simulink model "PV_MEV"  (R2025a)
settings: Solver=VariableStepAuto  StartTime=0.0  StopTime=10.0  RelTol=1e-3
InitFcn:
  | init_paras
values from neighbouring files (symbols this model uses):
  C_PFC = 2600e-6    (= 0.0026)    [init_paras.m]
  chg_ctrl_par = [Icc Vcv V_hys T_hys Kp_v_chg Ki_v_chg Kp_i_chg Ki_i_chg Ts_chg D_max_chg t_chg_on k_chg]    [init_paras.m]
  chg_ev = [0 Icc]    [init_paras.m]
  chg_par = [L_chg Voc Rint Ts_chg I_SIGN t_chg_on]    [init_paras.m]
  D = struct('X', {}, 'ti', {}, 'ia', {}, 'tc', {}, 'irms', {}, 'thd', {}, 'trip', {}, 'ttrip', {})    [make_waveform_figs.m]    (also in run_benchmark.m = get_sig('D'))
  det_ema_alpha = 0.1    [init_paras.m]
  det_force = 0    [init_paras.m]
  det_hyst = 0.6    [init_paras.m]
  det_persist = 2    [init_paras.m]
  det_src = 0    [init_paras.m]
  det_t_arm = 0.58    [init_paras.m]
  det_thr = [0.5 0.5 0.5 0.5 0.5]    [init_paras.m]
  det_variant_onehot = double(det_vlist == VARIANT_NAME)    [init_paras.m]
  ENABLE_HIL = 0    [init_paras.m]
  ENABLE_HIL_DET = 0    [init_paras.m]
  ENABLE_HIL_EST = 0    [init_paras.m]
  estimation_src = cfg_row.estimation_src    [init_paras.m]
  Fnom = 50    [init_paras.m]
  Fr_I = Fnom*2    (= 100)    [init_paras.m]
  grid_df = 0    [init_paras.m]
  grid_h5 = 0    [init_paras.m]
  grid_h7 = 0    [init_paras.m]
  grid_var_t0 = 0.7    [init_paras.m]
  hgq_fusion_alpha = [0.6704476522845647 0.7221651725151749 0.6446423751787858 0.41926421682656173]    [init_paras.m]
  hgq_min_ratio = single(0)    [init_paras.m]
  inj_channel = INJ.channel    [init_paras.m]
  inj_dwell = INJ.dwell    [init_paras.m]
  inj_shape = INJ.shape    [init_paras.m]
  inj_t_on = INJ.t_on    [init_paras.m]
  Ki_V = 80    [init_paras.m]
  Kp_I = 0.06    [init_paras.m]
  Kp_V = 0.25    [init_paras.m]
  Kr_I = 2.5    [init_paras.m]
  L_PFC = 600e-6    (= 0.0006)    [init_paras.m]
  Limit_V = 100    [init_paras.m]
  mit_t_ramp = 0.06    [init_paras.m]
  mitigation_mask = 0    [init_paras.m]
  mm_10cycle_points = mm_points_per_cycle * 10    (= 800)    [init_paras.m]
  mm_fund_freq = 50    [init_paras.m]
  mm_points_per_cycle = 80    [init_paras.m]
  R_bleed = 100e3    (= 100000)    [init_paras.m]
  R_pre = Ro*2    (= 44.44)    [init_paras.m]
  res_par = double(RES.par(:)'); end    [init_paras.m]
  RL_PFC = 20e-3    (= 0.02)    [init_paras.m]
  Ro = 22.22    [init_paras.m]
  t_pre_off = 0.30    (= 0.3)    [init_paras.m]
  Ts_chg = 10e-6    (= 1e-05)    [init_paras.m]
  Ts_Control = 1/Fc    [init_paras.m]
  Ts_Power = 50e-9    (= 5e-08)    [init_paras.m]    (also in run_benchmark.m = evalin('base','Ts_Power'))
  use_d_predict = cfg_row.use_d_predict    [init_paras.m]
  use_detector = 0    [init_paras.m]
  use_harmonic = cfg_row.use_harmonic    [init_paras.m]
  use_p_predict = cfg_row.use_p_predict    [init_paras.m]
  Vnom_ac = 240    [init_paras.m]
  vref_ev = [0 0]    [init_paras.m]
undefined symbols (not defined in the file or in its folder): D1, Delta, DiscIntNeverNeededParam
libraries: spsSeriesRLCBranchLib x17, spsMeanLib x16, MyLibrary x12, spsCurrentMeasurementLib x9, spsFourierLib x8, spsTHDLib x8, spsVoltageMeasurementLib x8, spsDiodeLib x7, simulink x7, pycoexlib x5, instrumentlib x4, spsPWMGeneratorDCDCLib x4
(part 5 of 7)

== system PV_MEV/PV System/DC DC Boost Converter ==
  note: 5 kHz - 500V
      | Boost Converter
  C1 : spsSeriesRLCBranchLib/Series RLC Branch  LConnTagsString=__new0  RConnTagsString=__new0  BranchType=C  Resistance=1.0  Inductance=1.0  SetiL0=off  InitialCurrent=0  Capacitance=12000e-06  Setx0=off  InitialVoltage=0  Measurements=None
  C2 : spsSeriesRLCBranchLib/Series RLC Branch  LConnTagsString=__new0  RConnTagsString=__new0  BranchType=C  Resistance=1.0  Inductance=1.0  SetiL0=off  InitialCurrent=0  Capacitance=12000e-06  Setx0=off  InitialVoltage=0  Measurements=None
  C3 : spsSeriesRLCBranchLib/Series RLC Branch  LConnTagsString=__new0  RConnTagsString=__new0  BranchType=C  Resistance=1.0  Inductance=1.0  SetiL0=off  InitialCurrent=0  Capacitance=100e-6  Setx0=off  InitialVoltage=0  Measurements=Branch voltage
  Deblock Converters : Step  Time=0.05  SampleTime=0
  Diode1 : spsDiodeLib/Diode  Ron=1e-4  Lon=0  Vf=0  IC=0  UseSnubber=off  Rs=inf  Cs=inf  Measurements=off
  Display : Display
  IGBT1 : spsIGBTLib/IGBT  Ron=0.001  Lon=0  Vf=0  Tf=0  Tt=0  IC=0  Rs=1e5  Cs=inf  Measurements=off
  L1 : spsSeriesRLCBranchLib/Series RLC Branch  LConnTagsString=__new0  RConnTagsString=__new0  BranchType=RL  Resistance=0.005  Inductance=5e-3  SetiL0=off  InitialCurrent=0  Capacitance=1e-6  Setx0=off  InitialVoltage=0  Measurements=None
  "MPPT Controller using  'Incremental Conductance + Integral Regulator'  technique " : Subsystem  mask(Boost Control - MPPT){fc=5000, T_MPPT=200e-6, Dinit=0.5}
      mask prompts: fc "PWM switching frequency (Hz)"; T_MPPT "Time window used by MPPT control (s)"; Dinit "Initial value of duty cycle"
  Product2 : Product  RndMeth=Zero
  "Vdc " : spsVoltageMeasurementLib/Voltage Measurement  Tag=PoWeRsYsTeMmEaSuReMeNt  PhasorSimulation=off  OutputType=Magnitude  PSBequivalent=0
  PV DC IN + : PMIOPort  Side=Left
  PV DC IN - : PMIOPort  Port=2  Side=Left
  BC DC OUT + : PMIOPort  Port=3  Side=Right
  BC DC MID : PMIOPort  Port=4  Side=Right
  BC DC OUT - : PMIOPort  Port=5  Side=Right
  tag scope: Vdc=global
  wires:
  Product2/1 -> IGBT1/1
  "Vdc "/1 -> Display/1, [Vdc]
  "MPPT Controller using  'Incremental Conductance + Integral Regulator'  technique "/1(Pulses) -> Product2/2
  Deblock Converters/1 -> Product2/1
  [V_PV] -> "MPPT Controller using  'Incremental Conductance + Integral Regulator'  technique "/1(V_PV)
  [I_PV] -> "MPPT Controller using  'Incremental Conductance + Integral Regulator'  technique "/2(I_PV)
  connections:
  Diode1/RConn1 -- "Vdc "/LConn1 -- C1/LConn1 -- BC DC OUT +/RConn1
  PV DC IN -/RConn1 -- C3/RConn1 -- IGBT1/RConn1 -- "Vdc "/LConn2 -- C2/RConn1 -- BC DC OUT -/RConn1
  L1/RConn1 -- Diode1/LConn1 -- IGBT1/LConn1
  C2/LConn1 -- C1/RConn1 -- BC DC MID/RConn1
  PV DC IN +/RConn1 -- C3/LConn1 -- L1/LConn1

== system PV_MEV/PV System/PV Enviroment ==
  Irradiance (W/m^2) : Display
  Irradiance Temp : SignalEditorBlockLib/Signal Editor  FileName=PVArrayGridData.mat  ActiveScenario=Ramp_up_down_Irradiance  ActiveSignal=Temp  IsBus=off  OutputBusObjectStr=Bus: BusObject  SampleTime=0  OutputAfterFinalValue=Extrapolation  Unit=inherit  PreserveSignalName=on  ApplySigPropsToAllScenarios=on  ApplySigPropsToAllSignals=off  SignalPropertySource=Dialog parameters
  Temperature (deg. C) : Display
  Ir : Outport
  Temp : Outport  Port=2
  wires:
  Irradiance Temp/1 -> Irradiance (W/m^2)/1, Ir/1
  ? -> Temperature (deg. C)/1, Temp/1

== system PV_MEV/PV System/PV Status ==
  m_PV : Inport
  Bus Selector : BusSelector  OutputSignals=V_PV,I_PV,I_diode,Irradiance (W/m2),Temperature (deg C)
  tag scope: I_PV=global, Idiode_PV=global, Ir=global, Temp=global, V_PV=global
  wires:
  Bus Selector/5 -> [Temp]  "<Temperature (deg C)>"
  Bus Selector/3 -> [Idiode_PV]  "<I_diode>"
  Bus Selector/2 -> [I_PV]  "<I_PV>"
  m_PV/1 -> Bus Selector/1
  Bus Selector/4 -> [Ir]  "<Irradiance (W/m2)>"
  Bus Selector/1 -> [V_PV]  "<V_PV>"

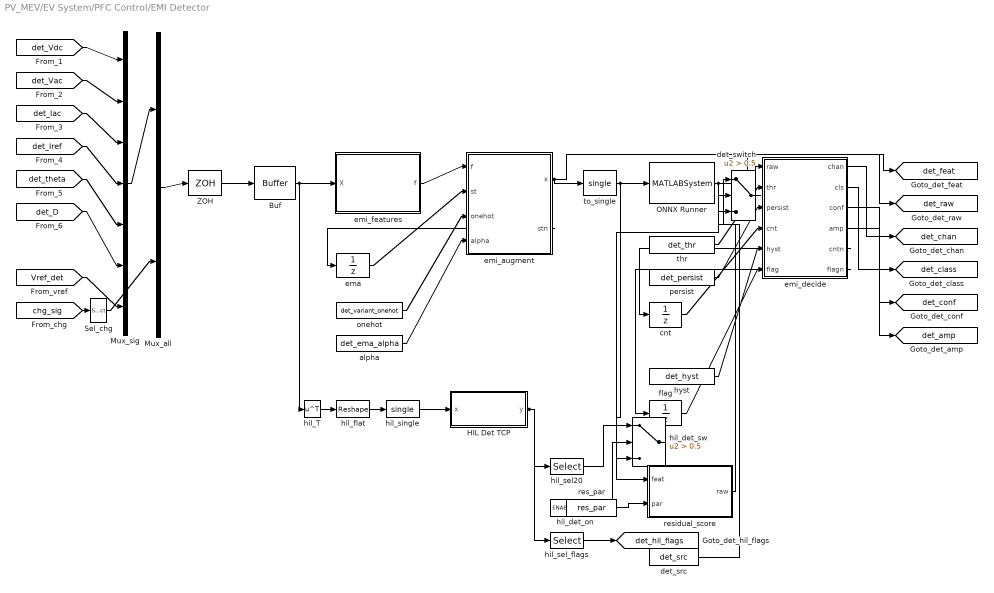
== system PV_MEV/EV System/PFC Control/EMI Detector ==
  Buf : Buffer  N=200
  HIL Det TCP : MATLAB Function  TreatAsAtomicUnit=on
  Mux_all : Mux  Inputs=2
  Mux_sig : Mux  Inputs=7
  ONNX Runner : MATLABSystem  System=OnnxRunner  ModelFile=/mnt/data6/playground/OLD_BRANCH/RL4EV/EMI_DET_FPGA/artifacts/detector.onnx  NumIn=48  NumOut=20  SampleTime=0.02
      mask Type: OnnxRunner
  Sel_chg : Selector  InputPortWidth=9  IndexOptions=Index vector (dialog)  Indices=[3 4 5 6 7]  OutputSizes=1
  ZOH : ZeroOrderHold  SampleTime=1e-4
  alpha : Constant  Value=det_ema_alpha
  cnt : UnitDelay  InitialCondition=zeros(1,5)  SampleTime=0.02  HasFrameUpgradeWarning=on
  det_src : Constant  Value=det_src
  det_switch : Switch  Criteria=u2 > Threshold  Threshold=0.5  SaturateOnIntegerOverflow=off  InputSameDT=off
  ema : UnitDelay  InitialCondition=zeros(1,49)  SampleTime=0.02  HasFrameUpgradeWarning=on
  emi_augment : MATLAB Function  TreatAsAtomicUnit=on
  emi_decide : MATLAB Function  TreatAsAtomicUnit=on
  emi_features : MATLAB Function  TreatAsAtomicUnit=on
  flag : UnitDelay  InitialCondition=zeros(1,5)  SampleTime=0.02  HasFrameUpgradeWarning=on
  hil_T : Math  Operator=transpose
  hil_det_on : Constant  Value=ENABLE_HIL_DET
  hil_det_sw : Switch  Criteria=u2 > Threshold  Threshold=0.5  SaturateOnIntegerOverflow=off  InputSameDT=off
  hil_flat : Reshape  OutputDimensionality=Row vector (2-D)
  hil_sel20 : Selector  InputPortWidth=21  IndexOptions=Index vector (dialog)  Indices=1:20  OutputSizes=1
  hil_sel_flags : Selector  InputPortWidth=21  IndexOptions=Index vector (dialog)  Indices=21  OutputSizes=1
  hil_single : DataTypeConversion  OutDataTypeStr=single  SaturateOnIntegerOverflow=off  RndMeth=Floor
  hyst : Constant  Value=det_hyst
  onehot : Constant  Value=det_variant_onehot
  persist : Constant  Value=det_persist
  res_par : Constant  Value=res_par
  residual_score : MATLAB Function  TreatAsAtomicUnit=on
  thr : Constant  Value=det_thr
  to_single : DataTypeConversion  OutDataTypeStr=single  SaturateOnIntegerOverflow=off  RndMeth=Floor
  tag scope: det_amp=global, det_chan=global, det_class=global, det_conf=global, det_feat=global, det_hil_flags=global, det_raw=global
  wires:
  [det_Vdc] -> Mux_sig/1
  [det_Vac] -> Mux_sig/2
  [det_Iac] -> Mux_sig/3
  [det_Iref] -> Mux_sig/4
  [det_theta] -> Mux_sig/5
  [det_D] -> Mux_sig/6
  [Vref_det] -> Mux_sig/7
  [chg_sig] -> Sel_chg/1
  Mux_sig/1 -> Mux_all/1
  Sel_chg/1 -> Mux_all/2
  Mux_all/1 -> ZOH/1
  ZOH/1 -> Buf/1
  Buf/1 -> emi_features/1(X), hil_T/1
  emi_features/1(f) -> emi_augment/1(f)
  ema/1 -> emi_augment/2(st)
  onehot/1 -> emi_augment/3(onehot)
  alpha/1 -> emi_augment/4(alpha)
  emi_augment/2(stn) -> ema/1
  emi_augment/1(x) -> to_single/1, [det_feat]
  to_single/1 -> ONNX Runner/1, residual_score/1(feat)
  ONNX Runner/1 -> [det_raw], hil_det_sw/3, det_switch/3
  thr/1 -> emi_decide/2(thr)
  persist/1 -> emi_decide/3(persist)
  cnt/1 -> emi_decide/4(cnt)
  hyst/1 -> emi_decide/5(hyst)
  flag/1 -> emi_decide/6(flag)
  emi_decide/5(cntn) -> cnt/1
  emi_decide/6(flagn) -> flag/1
  emi_decide/1(chan) -> [det_chan]
  emi_decide/2(cls) -> [det_class]
  emi_decide/3(conf) -> [det_conf]
  emi_decide/4(amp) -> [det_amp]
  hil_T/1 -> hil_flat/1
  hil_flat/1 -> hil_single/1
  hil_sel20/1 -> hil_det_sw/1
  hil_det_on/1 -> hil_det_sw/2
  hil_sel_flags/1 -> [det_hil_flags]
  hil_single/1 -> HIL Det TCP/1(x)
  HIL Det TCP/1(y) -> hil_sel20/1, hil_sel_flags/1
  res_par/1 -> residual_score/2(par)
  residual_score/1(raw) -> det_switch/1
  det_src/1 -> det_switch/2
  det_switch/1 -> emi_decide/1(raw)

== system PV_MEV/EV System/PFC Control/Enabled Subsystem ==
  Iac : Inport
  Data Type Conversion : DataTypeConversion  OutDataTypeStr=single  SaturateOnIntegerOverflow=off  RndMeth=Floor
  FFT Peak Hz : Display
  FFT Peak Receive : instrumentlib/TCP//IP Receive  Priority=20  Host=134.226.86.100  Port=5003  DataSize=[1, 1]  DataType=single  ASCIIFormatting=%f  Terminator=LF  CustomTerminator=10  ByteOrder=little-endian  EnableBlockingMode=on  Timeout=10  SampleTime=1/4000  SimulateUsing=Interpreted execution
  FFT TCP Send : instrumentlib/TCP//IP Send  Priority=-9  Host=134.226.86.100  Port=5002  ByteOrder=little-endian  EnableBlockingMode=on  Timeout=10  TransferDelay=off  SimulateUsing=Interpreted execution
  Scope1 : Scope  NumInputPorts=3
      settings: DataLoggingVariableName=ScopeData8  DataLoggingSaveFormat=Array
  TCP Sample Hold : ZeroOrderHold  SampleTime=1/4000
  TCP/IP Receive1 : instrumentlib/TCP//IP Receive  Priority=10  Host=134.226.86.100  Port=5001  DataSize=[1, 1]  DataType=single  ASCIIFormatting=%f  Terminator=LF  CustomTerminator=10  ByteOrder=little-endian  EnableBlockingMode=on  Timeout=10  SampleTime=1/4000  SimulateUsing=Interpreted execution
  TCP/IP Send1 : instrumentlib/TCP//IP Send  Priority=-10  Host=134.226.86.100  Port=5000  ByteOrder=little-endian  EnableBlockingMode=on  Timeout=10  TransferDelay=off  SimulateUsing=Interpreted execution
  wires:
  Data Type Conversion/1 -> Scope1/2, TCP/IP Send1/1, FFT TCP Send/1
  Iac/1 -> Scope1/1, TCP Sample Hold/1
  TCP Sample Hold/1 -> Data Type Conversion/1
  FFT Peak Receive/1 -> FFT Peak Hz/1
  TCP/IP Receive1/1 -> Scope1/3

== system PV_MEV/EV System/PFC Control/Half Cycle Model Prediction ==
  u : Inport
  Constant1 : Constant  Value=0.01
  Data Type Conversion : DataTypeConversion  SaturateOnIntegerOverflow=off  RndMeth=Floor
  Data Type Conversion1 : DataTypeConversion  SaturateOnIntegerOverflow=off  RndMeth=Floor
  Data Type Conversion2 : DataTypeConversion  SaturateOnIntegerOverflow=off  RndMeth=Floor
  Demux : Demux  Outputs=7
  MATLAB Function : MATLAB Function  TreatAsAtomicUnit=on
  MATLAB Function3 : MATLAB Function  TreatAsAtomicUnit=on
  Mux1 : Mux  Inputs=3
  Mux6 : Mux
  ONNX Model Predict : pycoexlib/ONNX Model Predict  ModelFile=/home/changhong/prj/finn_cli_fork/scripts/HIL/HarmonicAI_Simulation/Model_Training2/harmonic_brevitas_run_half_opt/brevitas_harmonic_mlp.onnx  ExecutionProviders=CPUExecutionProvider  InputTable={ 'input', 'float32', '', '2' }  OutputTable={ 'output', '', '' }  SampleTime=1/2000  InputDatatypes=float32  InputNumDims=2  InputPermutations=[]  OutputPermutations=[]  PythonCoexecutionBlockType=ONNXModelBlock  VariableOutputMaxSizes=[]
  Sampling1 : ZeroOrderHold  SampleTime=1/2000
  Transpose : Math  Operator=transpose
  u_buff : Buffer  N=40  V=39  OutputFrames=off
  amplitude : Outport
  phase : Outport  Port=2
  wires:
  Transpose/1 -> MATLAB Function/1(x)
  u_buff/1 -> Transpose/1
  u/1 -> Sampling1/1
  Mux1/1 -> phase/1
  Mux6/1 -> amplitude/1
  Data Type Conversion2/1 -> Demux/1
  MATLAB Function3/1(y_post) -> Data Type Conversion2/1
  Demux/1 -> Mux6/1
  Demux/2 -> Mux6/2
  Demux/3 -> Mux6/3
  Demux/4 -> Mux6/4
  Demux/5 -> Mux1/1
  Demux/6 -> Mux1/2
  Demux/7 -> Mux1/3
  MATLAB Function/2(A) -> MATLAB Function3/2(A_latest)
  Constant1/1 -> MATLAB Function3/3(alpha)
  Data Type Conversion1/1 -> MATLAB Function3/1(y_rel)
  ONNX Model Predict/1 -> Data Type Conversion1/1
  Data Type Conversion/1 -> ONNX Model Predict/1
  MATLAB Function/1(x_norm) -> Data Type Conversion/1
  Sampling1/1 -> u_buff/1

== system PV_MEV/EV System/PFC Control/One  Cycle Model Prediction ==
  u : Inport
  Constant1 : Constant
  Data Type Conversion : DataTypeConversion  SaturateOnIntegerOverflow=off  RndMeth=Floor
  Data Type Conversion1 : DataTypeConversion  SaturateOnIntegerOverflow=off  RndMeth=Floor
  Data Type Conversion2 : DataTypeConversion  SaturateOnIntegerOverflow=off  RndMeth=Floor
  Demux : Demux  Outputs=7
  HIL Est TCP : MATLAB Function  TreatAsAtomicUnit=on
  MATLAB Function : MATLAB Function  TreatAsAtomicUnit=on
  MATLAB Function3 : MATLAB Function  TreatAsAtomicUnit=on
  Mux1 : Mux  Inputs=3
  Mux6 : Mux
  ONNX Runner : MATLABSystem  System=OnnxRunner  ModelFile='D:/Prj/RL4EV/FFT_HGQ_BLS_FPGA/artifacts/harmonic_residual_bls_simulink.onnx'  NumIn=80  NumOut=8  SampleTime=1/(mm_fund_freq*mm_points_per_cycle)
      mask Type: OnnxRunner
  Sampling1 : ZeroOrderHold  SampleTime=1/(mm_fund_freq*mm_points_per_cycle)
  Transpose : Math  Operator=transpose
  hil_est_on : Constant  Value=ENABLE_HIL_EST
  hil_est_sw : Switch  Criteria=u2 > Threshold  Threshold=0.5  SaturateOnIntegerOverflow=off  InputSameDT=off
  hil_row : Reshape  OutputDimensionality=Row vector (2-D)
  hil_single : DataTypeConversion  OutDataTypeStr=single  SaturateOnIntegerOverflow=off  RndMeth=Floor
  u_buff : Buffer  N=mm_points_per_cycle  V=mm_sampling_overlap  OutputFrames=off
  amplitude : Outport
  phase : Outport  Port=2
  wires:
  Sampling1/1 -> u_buff/1
  MATLAB Function/1(x_norm) -> Data Type Conversion/1
  Data Type Conversion1/1 -> MATLAB Function3/1(y_encoded)
  Constant1/1 -> MATLAB Function3/3(ema_alpha)
  MATLAB Function/2(A) -> MATLAB Function3/2(window_peak)
  Demux/7 -> Mux1/3
  Demux/6 -> Mux1/2
  Demux/5 -> Mux1/1
  Demux/4 -> Mux6/4
  Demux/3 -> Mux6/3
  Demux/2 -> Mux6/2
  Demux/1 -> Mux6/1
  MATLAB Function3/1(y_post) -> Data Type Conversion2/1
  Data Type Conversion2/1 -> Demux/1
  Mux6/1 -> amplitude/1
  Mux1/1 -> phase/1
  u/1 -> Sampling1/1
  u_buff/1 -> Transpose/1
  Transpose/1 -> MATLAB Function/1(x), hil_single/1
  Data Type Conversion/1 -> ONNX Runner/1
  hil_single/1 -> hil_row/1
  hil_est_on/1 -> hil_est_sw/2
  ONNX Runner/1 -> hil_est_sw/3
  hil_est_sw/1 -> Data Type Conversion1/1
  hil_row/1 -> HIL Est TCP/1(x)
  HIL Est TCP/1(y) -> hil_est_sw/1

== system PV_MEV/EV System/PFC Control/PR2 ==
  Iref : Inport
  Iac : Inport  Port=2
  Gain : Gain  Gain=Kp
  Gain1 : Gain  Gain=Kr
  Second-Order Filter1 : spsSecondOrderFilterLib/Second-Order Filter  FilterType=Bandpass  Fo=Fr  Zeta=Zeta_I  Ts=Ts_Control  Initialize=off  Vac_Init="[0,  0,  60]"  Vdc_Init=0  PlotResponse=off  FreqRange=[0, 1000, 0.2]
  Sum1 : Sum  Inputs=|+-
  Sum2 : Sum  Inputs=|++
  D : Outport
  wires:
  Gain1/1 -> Second-Order Filter1/1
  Sum2/1 -> D/1
  Gain/1 -> Sum2/1
  Iac/1 -> Sum1/2
  Iref/1 -> Sum1/1
  Sum1/1 -> Gain1/1, Gain/1
  Second-Order Filter1/1 -> Sum2/2

== system PV_MEV/EV System/PFC Control/Speed Regulator2 ==
  note: Anti-windup mechanism: Method of conditionnal integration
      |
      | The integration is suspended if saturation occurs and the
      | control error is of the same sign as the control signal.
      |
      | [1] L.Rundqwist, "Anti-Reset Windup for PID Controllers," Ph.D. Thesis TRFT-1033,
      | Departement of Automatic Control, Lund Institute of Technology, Lund, Sweeden, 1991.
  Vref : Inport  PortDimensions=1
  Vmeas : Inport  Port=2  PortDimensions=1
  Ilim : Inport  Port=3
  Add : Sum  Inputs=+|-
  Compare To Zero : simulink/Logic and Bit Operations/Compare To Zero  relop=>  OutDataTypeStr=uint8  ZeroCross=off
  Compare To Zero1 : simulink/Logic and Bit Operations/Compare To Zero  relop=<  OutDataTypeStr=uint8  ZeroCross=off
  Constant : Constant  Value=0
  Discrete-Time Integrator : DiscreteIntegrator  IntegratorMethod=Integration: Trapezoidal  InitialCondition=Init  SampleTime=Ts  LimitOutput=on  UpperSaturationLimit=Limit_wreg  LowerSaturationLimit=-Limit_wreg  ShowStatePort=on  ICPrevOutput=DiscIntNeverNeededParam  ICPrevScaledInput=DiscIntNeverNeededParam
  Kp4 : Gain  Gain=Kp  SaturateOnIntegerOverflow=on  SampleTime=Ts  OutDataTypeStr=Inherit: Same as input  ParamDataTypeStr=Inherit: Same as input
  Kp5 : Gain  Gain=Ki  SaturateOnIntegerOverflow=on  SampleTime=Ts  OutDataTypeStr=Inherit: Same as input  ParamDataTypeStr=Inherit: Same as input
  Logical Operator : Logic  AllPortsSameDT=off  OutDataTypeStr=boolean
  Logical Operator1 : Logic  AllPortsSameDT=off  OutDataTypeStr=boolean
  Logical Operator2 : Logic  Operator=OR  AllPortsSameDT=off  OutDataTypeStr=boolean
  Relational Operator : RelationalOperator  OutDataTypeStr=boolean  InputSameDT=off
  Relational Operator1 : RelationalOperator  Operator=<=  OutDataTypeStr=boolean  InputSameDT=off
  SatDyn : simulink/Discontinuities/Saturation Dynamic  OutMin=[]  OutMax=[]  OutDataTypeStr=Inherit: Same as second input  OutDataType=fixdt(1, 16)  OutScaling=2^-10  DoSatur=off
  Sum1 : Sum  InputSameDT=on  SaturateOnIntegerOverflow=on  SampleTime=Ts  OutDataTypeStr=Inherit: Same as first input
  Sum6 : Sum  InputSameDT=on  SaturateOnIntegerOverflow=on  SampleTime=Ts  OutDataTypeStr=Inherit: Same as first input
  Switch : Switch  Criteria=u2 > Threshold  SaturateOnIntegerOverflow=off  InputSameDT=off
  Zero-Order Hold : ZeroOrderHold  SampleTime=Ts
  neg : Gain  Gain=-1
  Out : Outport  SampleTime=Ts  InitialOutput=0  VectorParamsAs1DForOutWhenUnconnected=off
  wires:
  Kp5/1 -> Switch/3
  Switch/1 -> Discrete-Time Integrator/1
  Discrete-Time Integrator/1 -> Sum6/2
  Kp4/1 -> Zero-Order Hold/1
  Add/1 -> Compare To Zero/1, Compare To Zero1/1, Kp5/1, Kp4/1
  Compare To Zero1/1 -> Logical Operator1/2  "Error_is_negative"
  Logical Operator1/1 -> Logical Operator2/2
  Logical Operator/1 -> Logical Operator2/1
  Compare To Zero/1 -> Logical Operator/2  "Error_is_positive"
  Relational Operator1/1 -> Logical Operator1/1  "LowerLimit_Is_Reached"
  Relational Operator/1 -> Logical Operator/1  "UpperLimit_is_Reached"
  Logical Operator2/1 -> Switch/2
  Sum1/1 -> Relational Operator/1, Relational Operator1/1
  Discrete-Time Integrator/State -> Sum1/1
  Zero-Order Hold/1 -> Sum6/1, Sum1/2
  Constant/1 -> Switch/1
  Vref/1 -> Add/1
  Vmeas/1 -> Add/2
  Ilim/1 -> Relational Operator/2, neg/1, SatDyn/1
  neg/1 -> Relational Operator1/2, SatDyn/3
  Sum6/1 -> SatDyn/2
  SatDyn/1 -> Out/1

== system PV_MEV/EV System/PFC Control/fft estimation 1 cycle2 ==
  u : Inport
  Buffer 1cycle : Buffer  N=mm_points_per_cycle  V=mm_sampling_overlap  OutputFrames=off
  Constant4 : Constant  Value=mm_fund_freq
  Constant5 : Constant  Value=mm_points_per_cycle * mm_fund_freq
  FFT_estimation_1 : MATLAB Function  TreatAsAtomicUnit=on
  Sampling : ZeroOrderHold  SampleTime=1/(mm_fund_freq*mm_points_per_cycle)
  amp : Outport
  phase : Outport  Port=2
  wires:
  Sampling/1 -> Buffer 1cycle/1
  Buffer 1cycle/1 -> FFT_estimation_1/1(u)
  Constant5/1 -> FFT_estimation_1/2(fs)
  Constant4/1 -> FFT_estimation_1/3(f0)
  u/1 -> Sampling/1
  FFT_estimation_1/1(amp) -> amp/1
  FFT_estimation_1/2(phase) -> phase/1

== system PV_MEV/EV System/PFC Control/fft estimation 10 cycle2 ==
  u : Inport
  Buffer 10cycle : Buffer  N=mm_10cycle_points  V=mm_10cycle_overlap  OutputFrames=off
  Constant4 : Constant  Value=mm_fund_freq
  Constant5 : Constant  Value=mm_points_per_cycle * mm_fund_freq
  FFT_estimation : MATLAB Function  TreatAsAtomicUnit=on
  Sampling : ZeroOrderHold  SampleTime=1/(mm_fund_freq*mm_points_per_cycle)
  amp : Outport
  phase : Outport  Port=2
  wires:
  FFT_estimation/2(phase) -> phase/1
  FFT_estimation/1(amp) -> amp/1
  u/1 -> Sampling/1
  Constant4/1 -> FFT_estimation/3(f0)
  Constant5/1 -> FFT_estimation/2(fs)
  Buffer 10cycle/1 -> FFT_estimation/1(u)
  Sampling/1 -> Buffer 10cycle/1

== system PV_MEV/EV System1/PFC Control/Half Cycle Model Prediction ==
  u : Inport
  Constant1 : Constant  Value=0.01
  Data Type Conversion : DataTypeConversion  SaturateOnIntegerOverflow=off  RndMeth=Floor
  Data Type Conversion1 : DataTypeConversion  SaturateOnIntegerOverflow=off  RndMeth=Floor
  Data Type Conversion2 : DataTypeConversion  SaturateOnIntegerOverflow=off  RndMeth=Floor
  Demux : Demux  Outputs=7
  MATLAB Function : MATLAB Function  TreatAsAtomicUnit=on
  MATLAB Function3 : MATLAB Function  TreatAsAtomicUnit=on
  Mux1 : Mux  Inputs=3
  Mux6 : Mux
  ONNX Model Predict : pycoexlib/ONNX Model Predict  ModelFile=/home/changhong/prj/finn_cli_fork/scripts/HIL/HarmonicAI_Simulation/Model_Training2/harmonic_brevitas_run_half_opt/brevitas_harmonic_mlp.onnx  ExecutionProviders=CPUExecutionProvider  InputTable={ 'input', 'float32', '', '2' }  OutputTable={ 'output', '', '' }  SampleTime=1/2000  InputDatatypes=float32  InputNumDims=2  InputPermutations=[]  OutputPermutations=[]  PythonCoexecutionBlockType=ONNXModelBlock  VariableOutputMaxSizes=[]
  Sampling1 : ZeroOrderHold  SampleTime=1/2000
  Transpose : Math  Operator=transpose
  u_buff : Buffer  N=40  V=39  OutputFrames=off
  amplitude : Outport
  phase : Outport  Port=2
  wires:
  Sampling1/1 -> u_buff/1
  MATLAB Function/1(x_norm) -> Data Type Conversion/1
  Data Type Conversion/1 -> ONNX Model Predict/1
  ONNX Model Predict/1 -> Data Type Conversion1/1
  Data Type Conversion1/1 -> MATLAB Function3/1(y_rel)
  Constant1/1 -> MATLAB Function3/3(alpha)
  MATLAB Function/2(A) -> MATLAB Function3/2(A_latest)
  Demux/7 -> Mux1/3
  Demux/6 -> Mux1/2
  Demux/5 -> Mux1/1
  Demux/4 -> Mux6/4
  Demux/3 -> Mux6/3
  Demux/2 -> Mux6/2
  Demux/1 -> Mux6/1
  MATLAB Function3/1(y_post) -> Data Type Conversion2/1
  Data Type Conversion2/1 -> Demux/1
  Mux6/1 -> amplitude/1
  Mux1/1 -> phase/1
  u/1 -> Sampling1/1
  u_buff/1 -> Transpose/1
  Transpose/1 -> MATLAB Function/1(x)

== system PV_MEV/EV System1/PFC Control/One  Cycle Model Prediction ==
  u : Inport
  Constant1 : Constant  Value=0.05
  Data Type Conversion : DataTypeConversion  SaturateOnIntegerOverflow=off  RndMeth=Floor
  Data Type Conversion1 : DataTypeConversion  SaturateOnIntegerOverflow=off  RndMeth=Floor
  Data Type Conversion2 : DataTypeConversion  SaturateOnIntegerOverflow=off  RndMeth=Floor
  Demux : Demux  Outputs=7
  MATLAB Function : MATLAB Function  TreatAsAtomicUnit=on
  MATLAB Function3 : MATLAB Function  TreatAsAtomicUnit=on
  Mux1 : Mux  Inputs=3
  Mux6 : Mux
  ONNX Model Predict : pycoexlib/ONNX Model Predict  ModelFile=/home/changhong/prj/finn_cli_fork/scripts/HIL/HarmonicAI_Simulation/Model_Training2/harmonic_brevitas_run_1cycle/brevitas_harmonic_mlp.onnx  ExecutionProviders=AzureExecutionProvider, CPUExecutionProvider  InputTable={ 'input', 'float32', '', '2' }  OutputTable={ 'output', '', '' }  SampleTime=1/4000  InputDatatypes=float32  InputNumDims=2  InputPermutations=[]  OutputPermutations=[]  PythonCoexecutionBlockType=ONNXModelBlock  VariableOutputMaxSizes=[]
  Sampling1 : ZeroOrderHold  SampleTime=1/(mm_fund_freq*mm_points_per_cycle)
  Transpose : Math  Operator=transpose
  u_buff : Buffer  N=mm_points_per_cycle  V=mm_sampling_overlap  OutputFrames=off
  amplitude : Outport
  phase : Outport  Port=2
  wires:
  Transpose/1 -> MATLAB Function/1(x)
  u_buff/1 -> Transpose/1
  u/1 -> Sampling1/1
  Mux1/1 -> phase/1
  Mux6/1 -> amplitude/1
  Data Type Conversion2/1 -> Demux/1
  MATLAB Function3/1(y_post) -> Data Type Conversion2/1
  Demux/1 -> Mux6/1
  Demux/2 -> Mux6/2
  Demux/3 -> Mux6/3
  Demux/4 -> Mux6/4
  Demux/5 -> Mux1/1
  Demux/6 -> Mux1/2
  Demux/7 -> Mux1/3
  MATLAB Function/2(A) -> MATLAB Function3/2(A_latest)
  Constant1/1 -> MATLAB Function3/3(alpha)
  Data Type Conversion1/1 -> MATLAB Function3/1(y_rel)
  ONNX Model Predict/1 -> Data Type Conversion1/1
  Data Type Conversion/1 -> ONNX Model Predict/1
  MATLAB Function/1(x_norm) -> Data Type Conversion/1
  Sampling1/1 -> u_buff/1

== system PV_MEV/EV System1/PFC Control/PR2 ==
  Iref : Inport
  Iac : Inport  Port=2
  Gain : Gain  Gain=Kp
  Gain1 : Gain  Gain=Kr
  Second-Order Filter1 : spsSecondOrderFilterLib/Second-Order Filter  FilterType=Bandpass  Fo=Fr  Zeta=Zeta_I  Ts=Ts_Control  Initialize=off  Vac_Init="[0,  0,  60]"  Vdc_Init=0  PlotResponse=off  FreqRange=[0, 1000, 0.2]
  Sum1 : Sum  Inputs=|+-
  Sum2 : Sum  Inputs=|++
  D : Outport
  wires:
  Second-Order Filter1/1 -> Sum2/2
  Sum1/1 -> Gain/1, Gain1/1
  Iref/1 -> Sum1/1
  Iac/1 -> Sum1/2
  Gain/1 -> Sum2/1
  Sum2/1 -> D/1
  Gain1/1 -> Second-Order Filter1/1

== system PV_MEV/EV System1/PFC Control/Speed Regulator2 ==
  note: Anti-windup mechanism: Method of conditionnal integration
      |
      | The integration is suspended if saturation occurs and the
      | control error is of the same sign as the control signal.
      |
      | [1] L.Rundqwist, "Anti-Reset Windup for PID Controllers," Ph.D. Thesis TRFT-1033,
      | Departement of Automatic Control, Lund Institute of Technology, Lund, Sweeden, 1991.
  Vref : Inport  PortDimensions=1
  Vmeas : Inport  Port=2  PortDimensions=1
  Add : Sum  Inputs=+|-
  Compare To Zero : simulink/Logic and Bit Operations/Compare To Zero  relop=>  OutDataTypeStr=uint8  ZeroCross=off
  Compare To Zero1 : simulink/Logic and Bit Operations/Compare To Zero  relop=<  OutDataTypeStr=uint8  ZeroCross=off
  Constant : Constant  Value=0
  Constant1 : Constant  Value=Limit_wreg
  Constant2 : Constant  Value=-Limit_wreg
  Discrete-Time Integrator : DiscreteIntegrator  IntegratorMethod=Integration: Trapezoidal  InitialCondition=Init  SampleTime=Ts  LimitOutput=on  UpperSaturationLimit=Limit_wreg  LowerSaturationLimit=-Limit_wreg  ShowStatePort=on  ICPrevOutput=DiscIntNeverNeededParam  ICPrevScaledInput=DiscIntNeverNeededParam
  Kp4 : Gain  Gain=Kp  SaturateOnIntegerOverflow=on  SampleTime=Ts  OutDataTypeStr=Inherit: Same as input  ParamDataTypeStr=Inherit: Same as input
  Kp5 : Gain  Gain=Ki  SaturateOnIntegerOverflow=on  SampleTime=Ts  OutDataTypeStr=Inherit: Same as input  ParamDataTypeStr=Inherit: Same as input
  Logical Operator : Logic  AllPortsSameDT=off  OutDataTypeStr=boolean
  Logical Operator1 : Logic  AllPortsSameDT=off  OutDataTypeStr=boolean
  Logical Operator2 : Logic  Operator=OR  AllPortsSameDT=off  OutDataTypeStr=boolean
  Relational Operator : RelationalOperator  OutDataTypeStr=boolean  InputSameDT=off
  Relational Operator1 : RelationalOperator  Operator=<=  OutDataTypeStr=boolean  InputSameDT=off
  Saturation2 : Saturate  UpperLimit=Limit_wreg  LowerLimit=-Limit_wreg  SampleTime=Ts
  Sum1 : Sum  InputSameDT=on  SaturateOnIntegerOverflow=on  SampleTime=Ts  OutDataTypeStr=Inherit: Same as first input
  Sum6 : Sum  InputSameDT=on  SaturateOnIntegerOverflow=on  SampleTime=Ts  OutDataTypeStr=Inherit: Same as first input
  Switch : Switch  Criteria=u2 > Threshold  SaturateOnIntegerOverflow=off  InputSameDT=off
  Zero-Order Hold : ZeroOrderHold  SampleTime=Ts
  Out : Outport  SampleTime=Ts  InitialOutput=0  VectorParamsAs1DForOutWhenUnconnected=off
  wires:
  Vmeas/1 -> Add/2
  Vref/1 -> Add/1
  Constant/1 -> Switch/1
  Zero-Order Hold/1 -> Sum1/2, Sum6/1
  Discrete-Time Integrator/State -> Sum1/1
  Sum1/1 -> Relational Operator1/1, Relational Operator/1
  Logical Operator2/1 -> Switch/2
  Relational Operator/1 -> Logical Operator/1  "UpperLimit_is_Reached"
  Relational Operator1/1 -> Logical Operator1/1  "LowerLimit_Is_Reached"
  Constant1/1 -> Relational Operator/2
  Constant2/1 -> Relational Operator1/2
  Compare To Zero/1 -> Logical Operator/2  "Error_is_positive"
  Logical Operator/1 -> Logical Operator2/1
  Logical Operator1/1 -> Logical Operator2/2
  Compare To Zero1/1 -> Logical Operator1/2  "Error_is_negative"
  Add/1 -> Kp4/1, Kp5/1, Compare To Zero1/1, Compare To Zero/1
  Sum6/1 -> Saturation2/1
  Kp4/1 -> Zero-Order Hold/1
  Discrete-Time Integrator/1 -> Sum6/2
  Saturation2/1 -> Out/1
  Switch/1 -> Discrete-Time Integrator/1
  Kp5/1 -> Switch/3

== system PV_MEV/EV System1/PFC Control/fft estimation 1 cycle2 ==
  u : Inport
  Buffer 1cycle : Buffer  N=mm_points_per_cycle  V=mm_sampling_overlap  OutputFrames=off
  Constant4 : Constant  Value=mm_fund_freq
  Constant5 : Constant  Value=mm_points_per_cycle * mm_fund_freq
  FFT_estimation_1 : MATLAB Function  TreatAsAtomicUnit=on
  Sampling : ZeroOrderHold  SampleTime=1/(mm_fund_freq*mm_points_per_cycle)
  amp : Outport
  phase : Outport  Port=2
  wires:
  FFT_estimation_1/2(phase) -> phase/1
  FFT_estimation_1/1(amp) -> amp/1
  u/1 -> Sampling/1
  Constant4/1 -> FFT_estimation_1/3(f0)
  Constant5/1 -> FFT_estimation_1/2(fs)
  Buffer 1cycle/1 -> FFT_estimation_1/1(u)
  Sampling/1 -> Buffer 1cycle/1

== system PV_MEV/EV System1/PFC Control/fft estimation 10 cycle2 ==
  u : Inport
  Buffer 10cycle : Buffer  N=mm_10cycle_points  V=mm_10cycle_overlap  OutputFrames=off
  Constant4 : Constant  Value=mm_fund_freq
  Constant5 : Constant  Value=mm_points_per_cycle * mm_fund_freq
  FFT_estimation : MATLAB Function  TreatAsAtomicUnit=on
  Sampling : ZeroOrderHold  SampleTime=1/(mm_fund_freq*mm_points_per_cycle)
  amp : Outport
  phase : Outport  Port=2
  wires:
  Sampling/1 -> Buffer 10cycle/1
  Buffer 10cycle/1 -> FFT_estimation/1(u)
  Constant5/1 -> FFT_estimation/2(fs)
  Constant4/1 -> FFT_estimation/3(f0)
  u/1 -> Sampling/1
  FFT_estimation/1(amp) -> amp/1
  FFT_estimation/2(phase) -> phase/1

== system PV_MEV/EV System2/PFC Control/Half Cycle Model Prediction ==
  u : Inport
  Constant1 : Constant  Value=0.01
  Data Type Conversion : DataTypeConversion  SaturateOnIntegerOverflow=off  RndMeth=Floor
  Data Type Conversion1 : DataTypeConversion  SaturateOnIntegerOverflow=off  RndMeth=Floor
  Data Type Conversion2 : DataTypeConversion  SaturateOnIntegerOverflow=off  RndMeth=Floor
  Demux : Demux  Outputs=7
  MATLAB Function : MATLAB Function  TreatAsAtomicUnit=on
  MATLAB Function3 : MATLAB Function  TreatAsAtomicUnit=on
  Mux1 : Mux  Inputs=3
  Mux6 : Mux
  ONNX Model Predict : pycoexlib/ONNX Model Predict  ModelFile=/home/changhong/prj/finn_cli_fork/scripts/HIL/HarmonicAI_Simulation/Model_Training2/harmonic_brevitas_run_half_opt/brevitas_harmonic_mlp.onnx  ExecutionProviders=CPUExecutionProvider  InputTable={ 'input', 'float32', '', '2' }  OutputTable={ 'output', '', '' }  SampleTime=1/2000  InputDatatypes=float32  InputNumDims=2  InputPermutations=[]  OutputPermutations=[]  PythonCoexecutionBlockType=ONNXModelBlock  VariableOutputMaxSizes=[]
  Sampling1 : ZeroOrderHold  SampleTime=1/2000
  Transpose : Math  Operator=transpose
  u_buff : Buffer  N=40  V=39  OutputFrames=off
  amplitude : Outport
  phase : Outport  Port=2
  wires:
  Transpose/1 -> MATLAB Function/1(x)
  u_buff/1 -> Transpose/1
  u/1 -> Sampling1/1
  Mux1/1 -> phase/1
  Mux6/1 -> amplitude/1
  Data Type Conversion2/1 -> Demux/1
  MATLAB Function3/1(y_post) -> Data Type Conversion2/1
  Demux/1 -> Mux6/1
  Demux/2 -> Mux6/2
  Demux/3 -> Mux6/3
  Demux/4 -> Mux6/4
  Demux/5 -> Mux1/1
  Demux/6 -> Mux1/2
  Demux/7 -> Mux1/3
  MATLAB Function/2(A) -> MATLAB Function3/2(A_latest)
  Constant1/1 -> MATLAB Function3/3(alpha)
  Data Type Conversion1/1 -> MATLAB Function3/1(y_rel)
  ONNX Model Predict/1 -> Data Type Conversion1/1
  Data Type Conversion/1 -> ONNX Model Predict/1
  MATLAB Function/1(x_norm) -> Data Type Conversion/1
  Sampling1/1 -> u_buff/1

== system PV_MEV/EV System2/PFC Control/One  Cycle Model Prediction ==
  u : Inport
  Constant1 : Constant  Value=0.05
  Data Type Conversion : DataTypeConversion  SaturateOnIntegerOverflow=off  RndMeth=Floor
  Data Type Conversion1 : DataTypeConversion  SaturateOnIntegerOverflow=off  RndMeth=Floor
  Data Type Conversion2 : DataTypeConversion  SaturateOnIntegerOverflow=off  RndMeth=Floor
  Demux : Demux  Outputs=7
  MATLAB Function : MATLAB Function  TreatAsAtomicUnit=on
  MATLAB Function3 : MATLAB Function  TreatAsAtomicUnit=on
  Mux1 : Mux  Inputs=3
  Mux6 : Mux
  ONNX Model Predict : pycoexlib/ONNX Model Predict  ModelFile=/home/changhong/prj/finn_cli_fork/scripts/HIL/HarmonicAI_Simulation/Model_Training2/harmonic_brevitas_run_1cycle/brevitas_harmonic_mlp.onnx  ExecutionProviders=AzureExecutionProvider, CPUExecutionProvider  InputTable={ 'input', 'float32', '', '2' }  OutputTable={ 'output', '', '' }  SampleTime=1/4000  InputDatatypes=float32  InputNumDims=2  InputPermutations=[]  OutputPermutations=[]  PythonCoexecutionBlockType=ONNXModelBlock  VariableOutputMaxSizes=[]
  Sampling1 : ZeroOrderHold  SampleTime=1/(mm_fund_freq*mm_points_per_cycle)
  Transpose : Math  Operator=transpose
  u_buff : Buffer  N=mm_points_per_cycle  V=mm_sampling_overlap  OutputFrames=off
  amplitude : Outport
  phase : Outport  Port=2
  wires:
  Sampling1/1 -> u_buff/1
  MATLAB Function/1(x_norm) -> Data Type Conversion/1
  Data Type Conversion/1 -> ONNX Model Predict/1
  ONNX Model Predict/1 -> Data Type Conversion1/1
  Data Type Conversion1/1 -> MATLAB Function3/1(y_rel)
  Constant1/1 -> MATLAB Function3/3(alpha)
  MATLAB Function/2(A) -> MATLAB Function3/2(A_latest)
  Demux/7 -> Mux1/3
  Demux/6 -> Mux1/2
  Demux/5 -> Mux1/1
  Demux/4 -> Mux6/4
  Demux/3 -> Mux6/3
  Demux/2 -> Mux6/2
  Demux/1 -> Mux6/1
  MATLAB Function3/1(y_post) -> Data Type Conversion2/1
  Data Type Conversion2/1 -> Demux/1
  Mux6/1 -> amplitude/1
  Mux1/1 -> phase/1
  u/1 -> Sampling1/1
  u_buff/1 -> Transpose/1
  Transpose/1 -> MATLAB Function/1(x)

== system PV_MEV/EV System2/PFC Control/PR2 ==
  Iref : Inport
  Iac : Inport  Port=2
  Gain : Gain  Gain=Kp
  Gain1 : Gain  Gain=Kr
  Second-Order Filter1 : spsSecondOrderFilterLib/Second-Order Filter  FilterType=Bandpass  Fo=Fr  Zeta=Zeta_I  Ts=Ts_Control  Initialize=off  Vac_Init="[0,  0,  60]"  Vdc_Init=0  PlotResponse=off  FreqRange=[0, 1000, 0.2]
  Sum1 : Sum  Inputs=|+-
  Sum2 : Sum  Inputs=|++
  D : Outport
  wires:
  Gain1/1 -> Second-Order Filter1/1
  Sum2/1 -> D/1
  Gain/1 -> Sum2/1
  Iac/1 -> Sum1/2
  Iref/1 -> Sum1/1
  Sum1/1 -> Gain1/1, Gain/1
  Second-Order Filter1/1 -> Sum2/2

== system PV_MEV/EV System2/PFC Control/Speed Regulator2 ==
  note: Anti-windup mechanism: Method of conditionnal integration
      |
      | The integration is suspended if saturation occurs and the
      | control error is of the same sign as the control signal.
      |
      | [1] L.Rundqwist, "Anti-Reset Windup for PID Controllers," Ph.D. Thesis TRFT-1033,
      | Departement of Automatic Control, Lund Institute of Technology, Lund, Sweeden, 1991.
  Vref : Inport  PortDimensions=1
  Vmeas : Inport  Port=2  PortDimensions=1
  Add : Sum  Inputs=+|-
  Compare To Zero : simulink/Logic and Bit Operations/Compare To Zero  relop=>  OutDataTypeStr=uint8  ZeroCross=off
  Compare To Zero1 : simulink/Logic and Bit Operations/Compare To Zero  relop=<  OutDataTypeStr=uint8  ZeroCross=off
  Constant : Constant  Value=0
  Constant1 : Constant  Value=Limit_wreg
  Constant2 : Constant  Value=-Limit_wreg
  Discrete-Time Integrator : DiscreteIntegrator  IntegratorMethod=Integration: Trapezoidal  InitialCondition=Init  SampleTime=Ts  LimitOutput=on  UpperSaturationLimit=Limit_wreg  LowerSaturationLimit=-Limit_wreg  ShowStatePort=on  ICPrevOutput=DiscIntNeverNeededParam  ICPrevScaledInput=DiscIntNeverNeededParam
  Kp4 : Gain  Gain=Kp  SaturateOnIntegerOverflow=on  SampleTime=Ts  OutDataTypeStr=Inherit: Same as input  ParamDataTypeStr=Inherit: Same as input
  Kp5 : Gain  Gain=Ki  SaturateOnIntegerOverflow=on  SampleTime=Ts  OutDataTypeStr=Inherit: Same as input  ParamDataTypeStr=Inherit: Same as input
  Logical Operator : Logic  AllPortsSameDT=off  OutDataTypeStr=boolean
  Logical Operator1 : Logic  AllPortsSameDT=off  OutDataTypeStr=boolean
  Logical Operator2 : Logic  Operator=OR  AllPortsSameDT=off  OutDataTypeStr=boolean
  Relational Operator : RelationalOperator  OutDataTypeStr=boolean  InputSameDT=off
  Relational Operator1 : RelationalOperator  Operator=<=  OutDataTypeStr=boolean  InputSameDT=off
  Saturation2 : Saturate  UpperLimit=Limit_wreg  LowerLimit=-Limit_wreg  SampleTime=Ts
  Sum1 : Sum  InputSameDT=on  SaturateOnIntegerOverflow=on  SampleTime=Ts  OutDataTypeStr=Inherit: Same as first input
  Sum6 : Sum  InputSameDT=on  SaturateOnIntegerOverflow=on  SampleTime=Ts  OutDataTypeStr=Inherit: Same as first input
  Switch : Switch  Criteria=u2 > Threshold  SaturateOnIntegerOverflow=off  InputSameDT=off
  Zero-Order Hold : ZeroOrderHold  SampleTime=Ts
  Out : Outport  SampleTime=Ts  InitialOutput=0  VectorParamsAs1DForOutWhenUnconnected=off
  wires:
  Kp5/1 -> Switch/3
  Switch/1 -> Discrete-Time Integrator/1
  Saturation2/1 -> Out/1
  Discrete-Time Integrator/1 -> Sum6/2
  Kp4/1 -> Zero-Order Hold/1
  Sum6/1 -> Saturation2/1
  Add/1 -> Compare To Zero/1, Compare To Zero1/1, Kp5/1, Kp4/1
  Compare To Zero1/1 -> Logical Operator1/2  "Error_is_negative"
  Logical Operator1/1 -> Logical Operator2/2
  Logical Operator/1 -> Logical Operator2/1
  Compare To Zero/1 -> Logical Operator/2  "Error_is_positive"
  Constant2/1 -> Relational Operator1/2
  Constant1/1 -> Relational Operator/2
  Relational Operator1/1 -> Logical Operator1/1  "LowerLimit_Is_Reached"
  Relational Operator/1 -> Logical Operator/1  "UpperLimit_is_Reached"
  Logical Operator2/1 -> Switch/2
  Sum1/1 -> Relational Operator/1, Relational Operator1/1
  Discrete-Time Integrator/State -> Sum1/1
  Zero-Order Hold/1 -> Sum6/1, Sum1/2
  Constant/1 -> Switch/1
  Vref/1 -> Add/1
  Vmeas/1 -> Add/2

== system PV_MEV/EV System2/PFC Control/fft estimation 1 cycle2 ==
  u : Inport
  Buffer 1cycle : Buffer  N=mm_points_per_cycle  V=mm_sampling_overlap  OutputFrames=off
  Constant4 : Constant  Value=mm_fund_freq
  Constant5 : Constant  Value=mm_points_per_cycle * mm_fund_freq
  FFT_estimation_1 : MATLAB Function  TreatAsAtomicUnit=on
  Sampling : ZeroOrderHold  SampleTime=1/(mm_fund_freq*mm_points_per_cycle)
  amp : Outport
  phase : Outport  Port=2
  wires:
  Sampling/1 -> Buffer 1cycle/1
  Buffer 1cycle/1 -> FFT_estimation_1/1(u)
  Constant5/1 -> FFT_estimation_1/2(fs)
  Constant4/1 -> FFT_estimation_1/3(f0)
  u/1 -> Sampling/1
  FFT_estimation_1/1(amp) -> amp/1
  FFT_estimation_1/2(phase) -> phase/1

== system PV_MEV/EV System2/PFC Control/fft estimation 10 cycle2 ==
  u : Inport
  Buffer 10cycle : Buffer  N=mm_10cycle_points  V=mm_10cycle_overlap  OutputFrames=off
  Constant4 : Constant  Value=mm_fund_freq
  Constant5 : Constant  Value=mm_points_per_cycle * mm_fund_freq
  FFT_estimation : MATLAB Function  TreatAsAtomicUnit=on
  Sampling : ZeroOrderHold  SampleTime=1/(mm_fund_freq*mm_points_per_cycle)
  amp : Outport
  phase : Outport  Port=2
  wires:
  FFT_estimation/2(phase) -> phase/1
  FFT_estimation/1(amp) -> amp/1
  u/1 -> Sampling/1
  Constant4/1 -> FFT_estimation/3(f0)
  Constant5/1 -> FFT_estimation/2(fs)
  Buffer 10cycle/1 -> FFT_estimation/1(u)
  Sampling/1 -> Buffer 10cycle/1

== system PV_MEV/PV System/DC AC Inverter/VSC Control ==
  note: VSC Main Controller
  Vabc_prim : Inport  PortDimensions=3
  Iabc_prim : Inport  Port=2  PortDimensions=3
  Vdc_mes : Inport  Port=3  PortDimensions=1
  Current Regulator : Subsystem
  Iq_ref : Constant  Value=0
  Mux : Mux  Inputs=2
  PLL & Measurements : Subsystem
  PWM Generator (3-Level) : spsPWMGenerator3LevelLib/PWM Generator (3-Level)  ModulatorType=Three-phase bridge (12 pulses)  ModulatorMode=Unsynchronized  nF=27  Fc=33*60  ModulatingSignals=off  m=0.8  Freq=60  Phase=0  Ts=Ts_Power
  Uabc_ref Generation max (m) = 1 : Subsystem
  Unit Delay : UnitDelay  SampleTime=Ts_Control  HasFrameUpgradeWarning=on
  VDC Regulator : Subsystem
  Vdc_ref1 : Constant  Value=Vdc_ref
  Pulses : Outport  VectorParamsAs1DForOutWhenUnconnected=off
  wires:
  VDC Regulator/1(Id_ref) -> Mux/1
  PLL & Measurements/1(wt) -> Uabc_ref Generation max (m) = 1/1(wt)
  Current Regulator/1(VdVq_conv) -> Uabc_ref Generation max (m) = 1/2(VdVq_conv)
  Iq_ref/1 -> Mux/2
  Mux/1 -> Current Regulator/3(IdIq_ref)
  PLL & Measurements/3(IdIq_prim) -> Current Regulator/2(IdIq_mes)
  PLL & Measurements/2(VdVq_prim) -> Current Regulator/1(VdVq_mes)
  Vdc_mes/1 -> VDC Regulator/1(Vdc_mes)
  Vabc_prim/1 -> PLL & Measurements/1(Vabc_prim)
  Iabc_prim/1 -> PLL & Measurements/2(Iabc_prim)
  Unit Delay/1 -> PWM Generator (3-Level)/1
  PWM Generator (3-Level)/1 -> Pulses/1
  Uabc_ref Generation max (m) = 1/1(Uabc_ref) -> Unit Delay/1
  Vdc_ref1/1 -> VDC Regulator/2(Vdc_ref)

== system PV_MEV/PV System/DC DC Boost Converter/MPPT Controller using  'Incremental Conductance + Integral Regulator'  technique  ==
  V_PV : Inport
  I_PV : Inport  Port=2
  Add : Sum  Inputs=+-
  Deblock MPPT : Step  Time=0.4  SampleTime=0
  Duty Cycle : Constant  Value=Dinit
  MPPT : Subsystem
  PWM Generator (DC-DC) : spsPWMGeneratorDCDCLib/PWM Generator (DC-DC)  Fsw=fc  Ts=Ts_Power
  Saturation : Saturate  UpperLimit=1  LowerLimit=0
  Pulses : Outport  VectorParamsAs1DForOutWhenUnconnected=off
  tag scope: D=global
  wires:
  V_PV/1 -> MPPT/1(V_PV)
  I_PV/1 -> MPPT/2(I_PV)
  PWM Generator (DC-DC)/1 -> Pulses/1
  Deblock MPPT/1 -> MPPT/3(on/off)
  Saturation/1 -> PWM Generator (DC-DC)/1, [D]
  Add/1 -> Saturation/1  "D"
  MPPT/1(Delta_D) -> Add/2
  Duty Cycle/1 -> Add/1

== system PV_MEV/PV System/DC AC Inverter/VSC Control/Current Regulator ==
  note: harmonic filter neglected
  note: Vd_mes + Id*R - Iq*L + deriv(Id)*L= Vd_conv
  note: Vq_mes + Id*L + Iq*R + deriv(Iq)*L= Vq_conv
  note: Current Regulator
      | (with feedforward)
  note: Sign Convention: Current going out of the converter = positive current
  note: Iq positive --> The converter absorbs reactive power ("Inductive mode") = Reactive Power Q negative
  note: Id positive --> The converter generates active power ("Inverter mode") = Active Power P positive
  note: Ltot = Lxfo + Lchoke
      | Rtot = Rxfo + Rchoke
  note: (Vd_prim - Vd_conv) ~= + Iq * Ltot
  note: (Vq_prim - Vq_conv) ~ = - Id * Ltot
  note: For Ltot >> Rtot :
  VdVq_mes : Inport  PortDimensions=2
  IdIq_mes : Inport  Port=2  PortDimensions=2
  IdIq_ref : Inport  Port=3  PortDimensions=2
  Add1 : Sum  Inputs=++-
  Add2 : Sum
  Add3 : Sum  Inputs=+++
  Demux : Demux  Outputs=2
  Demux1 : Demux  Outputs=2
  Ltot_pu1 : Gain  Gain=Ltot_pu  SaturateOnIntegerOverflow=on  OutDataTypeStr=Inherit: Same as input  ParamDataTypeStr=Inherit: Same as input
  Ltot_pu2 : Gain  Gain=Ltot_pu  SaturateOnIntegerOverflow=on  OutDataTypeStr=Inherit: Same as input  ParamDataTypeStr=Inherit: Same as input
  Mux : Mux  Inputs=2
  PI : slpidlib/PID Controller  Controller=PI  Form=Parallel  TimeDomain=Discrete-time  UseExternalTs=off  SampleTime=Ts  IntegratorMethod=Forward Euler  FilterMethod=Forward Euler  ControllerParametersSource=internal  P=Kp_Ireg  I=Ki_Ireg  UseKiTs=off  D=0  UseExternalDerivativeSource=off  N=100  UseFilter=on  TunerSelectOption=Transfer Function Based (PID Tuner App)  InitialConditionSource=internal  InitialConditionForIntegrator=0  InitialConditionForFilter=0  DifferentiatorICPrevScaledInput=0  ExternalReset=none  TrackingMode=off  Kt=1  LimitOutput=on  SatLimitsSource=internal  UpperSaturationLimit=2  LowerSaturationLimit=-2  LinearizeAsGain=off  AntiWindupMode=none  Kb=1  LimitIntegrator=off  UpperIntegratorSaturationLimit=inf  LowerIntegratorSaturationLimit=-inf  POutMin=[]  POutMax=[]  IOutMin=[]  IOutMax=[]  DOutMin=[]  DOutMax=[]  NOutMin=[]  NOutMax=[]  SumOutMin=[]  SumOutMax=[]  SaturationOutMin=[]  SaturationOutMax=[]  PParamMin=[]  PParamMax=[]  IParamMin=[]  IParamMax=[]  DParamMin=[]  DParamMax=[]  NParamMin=[]  NParamMax=[]  KbParamMin=[]  KbParamMax=[]  KtParamMin=[]  KtParamMax=[]  KbOutMin=[]  KbOutMax=[]  KtOutMin=[]  KtOutMax=[]  IntegratorOutMin=[]  IntegratorOutMax=[]  FilterOutMin=[]  FilterOutMax=[]  SumI1OutMin=[]  SumI1OutMax=[]  SumI2OutMin=[]  SumI2OutMax=[]  SumI3OutMin=[]  SumI3OutMax=[]  SumI4OutMin=[]  SumI4OutMax=[]  SumDOutMin=[]  SumDOutMax=[]  DifferentiatorOutMin=[]  DifferentiatorOutMax=[]  FilterDiffOutCoefMin=[]  FilterDiffOutCoefMax=[]  ReciprocalOutMin=[]  ReciprocalOutMax=[]  SumDenOutMin=[]  SumDenOutMax=[]  SumNumOutMin=[]  SumNumOutMax=[]  DivideOutMin=[]  DivideOutMax=[]  UdiffTsProdOutMin=[]  UdiffTsProdOutMax=[]  NTsProdOutMin=[]  NTsProdOutMax=[]  UintegralTsProdOutMin=[]  UintegralTsProdOutMax=[]  UngainTsProdOutMin=[]  UngainTsProdOutMax=[]  ClampingZeroOutDataTypeStr=Inherit: Inherit via back propagation  ClampingZeroOutMin=[]  ClampingZeroOutMax=[]  FilterDenConstantOutDataTypeStr=Inherit: Inherit via back propagation  FilterDenConstantOutMin=[]  FilterDenConstantOutMax=[]  PCopyOutDataTypeStr=Inherit: Inherit via back propagation  PCopyOutMin=[]  PCopyOutMax=[]  NCopyOutDataTypeStr=Inherit: Inherit via back propagation  NCopyOutMin=[]  NCopyOutMax=[]  IntegratorContinuousStateAttributes=''  IntegratorStateMustResolveToSignalObject=off  IntegratorRTWStateStorageClass=Auto  FilterContinuousStateAttributes=''  FilterStateMustResolveToSignalObject=off  FilterRTWStateStorageClass=Auto  ParallelPVariant=InternalParameters  IdealPVariant=Disabled  IVariant=InternalParameters  DVariant=Disabled  IntegratorVariant=Discrete  SatVariant=Enabled  AWVariant=Passthrough  PCopyVariant=Disabled  TRVariant=Disabled  FdbkBlocksVariant=Forward  IdealPFdbkVariant=Disabled  SatFdbkVariant=Disabled  DerivativeFilterVariant=Disabled  NVariant=Disabled  NCopyVariant=Disabled_SignalSpec  FilterICVariant=Disabled  IntegratorICVariant=InternalICs  ExternalResetVariant=Disabled  TRSumVariant=Passthrough  SumFdbkVariant=Disabled  SumVariant=Sum_PI  TsampFilterVariant=InternalTs  TsampNgainVariant=Passthrough  TsampIntegralVariant=Disabled_SignalSpec  ExternalSaturationOutDataTypeStr=Inherit: Same as second input  DerivativeSourceVariant=Disabled  PreIntVariant=InternalPreInt
  PI_Ireg1 : Scope
      settings: DataLoggingSaveFormat=Array
  Rtot_pu1 : Gain  Gain=Rtot_pu  SaturateOnIntegerOverflow=on  OutDataTypeStr=Inherit: Same as input  ParamDataTypeStr=Inherit: Same as input
  Rtot_pu5 : Gain  Gain=Rtot_pu  SaturateOnIntegerOverflow=on  OutDataTypeStr=Inherit: Same as input  ParamDataTypeStr=Inherit: Same as input
  Saturation : Saturate  UpperLimit=2  LowerLimit=-2
  Sum : Sum  Inputs=|-+
  VdVq_conv : Outport  VectorParamsAs1DForOutWhenUnconnected=off
  wires:
  Mux/1 -> PI_Ireg1/1, Add2/2
  PI/1 -> Add2/1  "PI"
  Sum/1 -> PI/1
  IdIq_ref/1 -> Sum/2, Demux1/1
  IdIq_mes/1 -> Sum/1
  Add2/1 -> Saturation/1
  Saturation/1 -> VdVq_conv/1
  VdVq_mes/1 -> Demux/1
  Demux/1 -> Add1/1
  Rtot_pu1/1 -> Add1/2
  Demux1/1 -> Rtot_pu1/1, Ltot_pu2/1
  Ltot_pu1/1 -> Add1/3
  Demux1/2 -> Ltot_pu1/1, Rtot_pu5/1
  Rtot_pu5/1 -> Add3/2
  Ltot_pu2/1 -> Add3/3
  Add1/1 -> Mux/1  "Feedforward"
  Demux/2 -> Add3/1
  Add3/1 -> Mux/2
